simulink model "EarlyReturn11_2018a"  (R2018a)
settings: Solver=VariableStepAuto  StartTime=0.0  StopTime=0.2  RelTol=1e-3
settings Model: Creator=BEAR  LastModifiedBy=bzhan

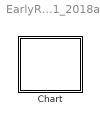
== system EarlyReturn11_2018a ==
  Chart : Stateflow chart  TreatAsAtomicUnit=on

== stateflow chart EarlyReturn11_2018a/Chart ==
  settings: updateMethod=DISCRETE  sampleTime=0.1
  state A
    en: f("en_A")
    ex: f("ex_A")
    state A2
      en: f("en_A2")
      ex: f("ex_A2")
      state A2a
        en: f("en_A2a")
        ex: f("ex_A2a")
    state A3
      en: f("en_A3")
      ex: f("ex_A3")
      state A3a
        en: f("en_A3a")
        ex: f("ex_A3a")
    state A1
      en: f("en_A1")
      ex: f("ex_A1")
    (default) -> A1
    A1 -> A2a
    A2a -> A3a : /{E;f("ta")}
  (default) -> A
  A -> A : E{f("loop")}
  data: s function_input
  events: E local FUNCTION_CALL_EVENT
  function f(s):
    | function f(s)
    |   fprintf(s+"\n");
